simulink model "ieee80211n"  (Simulink 6.0)
settings: Solver=VariableStepDiscrete  StartTime=0.0  StopTime=inf  RelTol=1e-3
PreLoadFcn:
  | load IEEE80211n_init;
values from neighbouring files (symbols this model uses):
  params =     [IEEE80211n_init.mat]    (also in IEEE80211n_settings.m = p)
undefined symbols (not defined in the file or in its folder): magnitude
libraries: commblkintrlv2 x196, dspsigops x143, simulink x136, commdigbbndam2 x98, dspmtrx3 x96, dspsigattribs x69, dspstat3 x38, commutil2 x32, commsequence2 x26, commcnvcod2 x10, dspindex x9, dspmlti3 x8
(part 8 of 12)

== system ieee80211n/Demodbank/Demod_ss3/Demodulator 4 ==
  rxsig : Inport  Port=1  LatchInput=off
  mscale : Inport  Port=2  LatchInput=off
  Enable : EnablePort
  Bits Per Symbol : Constant  Value=ones(1, log2(modOrder))  VectorParams1D=off
  General Block Deinterleaver : commblkintrlv2/General Block Deinterleaver  elements=interleaverElements
  General Block Deinterleaver1 : S-Function  AncestorBlock=commblkintrlv2/General Block Deinterleaver  FunctionName=scominterl  Parameters=elements,method  mask(General Block Deinterleaver){elements=freqRotInterleaverElements}
      mask help: Reorder the elements of the input vector. y(elements) = u. The length of Elements must match the input signal width.
      mask init:
      | method = 2;
      | commblkinterl(elements);
      mask Help: helpview(commbhelp)
      mask Display: disp('Frequency\nRotation\nDeinterleaver')
  General Block Deinterleaver2 : commblkintrlv2/General Block Deinterleaver  elements=interleaverElements
  General Block Deinterleaver3 : S-Function  AncestorBlock=commblkintrlv2/General Block Deinterleaver  FunctionName=scominterl  Parameters=elements,method  mask(General Block Deinterleaver){elements=freqRotInterleaverElements}
      mask help: Reorder the elements of the input vector. y(elements) = u. The length of Elements must match the input signal width.
      mask init:
      | method = 2;
      | commblkinterl(elements);
      mask Help: helpview(commbhelp)
      mask Display: disp('Frequency\nRotation\nDeinterleaver')
  Matrix Deinterleaver : commblkintrlv2/Matrix Deinterleaver  Nrows=interleaverRows  Ncols=interleaverCols
  Matrix Deinterleaver1 : commblkintrlv2/Matrix Deinterleaver  Nrows=interleaverRows  Ncols=interleaverCols
  Matrix Multiply : Product  Multiplication=Matrix(*)
  Rectangular QAM Demodulator Baseband : commdigbbndam2/Rectangular QAM Demodulator Baseband  M=modOrder  OutType=Bit  Dec=Gray  PowType=Average Power  MinDist=2  AvgPow=1  PeakPow=1  Ph=0  numSamp=1
  Rectangular QAM Modulator Baseband1 : commdigbbndam2/Rectangular QAM Modulator Baseband  M=modOrder  InType=Bit  Enc=Gray  PowType=Average Power  MinDist=2  AvgPow=1  PeakPow=1  Ph=0  numSamp=1
  Reshape6 : simulink/Math Operations/Reshape  OutputDimensionality=Column vector  OutputDimensions=1600
  Sum : Sum  Inputs=|+-  SaturateOnIntegerOverflow=on
  Transpose : dspmtrx3/Transpose  Hermitian=off  overflowFlag=on
  Unipolar to Bipolar Converter2 : commutil2/Unipolar to Bipolar Converter  M=2  polarity=Negative
  rxdata : Outport  OutputWhenDisabled=reset  InitialOutput=0
  symerr : Outport  Port=2  OutputWhenDisabled=reset  InitialOutput=0
  mscale out : Outport  Port=3  OutputWhenDisabled=reset  InitialOutput=0
  wires:
  General Block Deinterleaver/1 -> Matrix Deinterleaver/1
  Matrix Deinterleaver/1 -> rxdata/1
  Sum/1 -> symerr/1
  Rectangular QAM Modulator Baseband1/1 -> Sum/1
  Unipolar to Bipolar Converter2/1 -> General Block Deinterleaver1/1
  rxsig/1 -> Sum/2, Rectangular QAM Demodulator Baseband/1
  Rectangular QAM Demodulator Baseband/1 -> Rectangular QAM Modulator Baseband1/1, Unipolar to Bipolar Converter2/1
  General Block Deinterleaver1/1 -> General Block Deinterleaver/1
  mscale/1 -> Matrix Multiply/1
  Matrix Multiply/1 -> Transpose/1
  Bits Per Symbol/1 -> Matrix Multiply/2
  Reshape6/1 -> General Block Deinterleaver3/1
  Transpose/1 -> Reshape6/1
  General Block Deinterleaver2/1 -> Matrix Deinterleaver1/1
  Matrix Deinterleaver1/1 -> mscale out/1
  General Block Deinterleaver3/1 -> General Block Deinterleaver2/1

== system ieee80211n/Demodbank/Demod_ss3/Demodulator 5 ==
  rxsig : Inport  Port=1  LatchInput=off
  mscale : Inport  Port=2  LatchInput=off
  Enable : EnablePort
  Bits Per Symbol : Constant  Value=ones(1, log2(modOrder))  VectorParams1D=off
  General Block Deinterleaver : commblkintrlv2/General Block Deinterleaver  elements=interleaverElements
  General Block Deinterleaver1 : S-Function  AncestorBlock=commblkintrlv2/General Block Deinterleaver  FunctionName=scominterl  Parameters=elements,method  mask(General Block Deinterleaver){elements=freqRotInterleaverElements}
      mask help: Reorder the elements of the input vector. y(elements) = u. The length of Elements must match the input signal width.
      mask init:
      | method = 2;
      | commblkinterl(elements);
      mask Help: helpview(commbhelp)
      mask Display: disp('Frequency\nRotation\nDeinterleaver')
  General Block Deinterleaver2 : commblkintrlv2/General Block Deinterleaver  elements=interleaverElements
  General Block Deinterleaver3 : S-Function  AncestorBlock=commblkintrlv2/General Block Deinterleaver  FunctionName=scominterl  Parameters=elements,method  mask(General Block Deinterleaver){elements=freqRotInterleaverElements}
      mask help: Reorder the elements of the input vector. y(elements) = u. The length of Elements must match the input signal width.
      mask init:
      | method = 2;
      | commblkinterl(elements);
      mask Help: helpview(commbhelp)
      mask Display: disp('Frequency\nRotation\nDeinterleaver')
  Matrix Deinterleaver : commblkintrlv2/Matrix Deinterleaver  Nrows=interleaverRows  Ncols=interleaverCols
  Matrix Deinterleaver1 : commblkintrlv2/Matrix Deinterleaver  Nrows=interleaverRows  Ncols=interleaverCols
  Matrix Multiply : Product  Multiplication=Matrix(*)
  Rectangular QAM Demodulator Baseband : commdigbbndam2/Rectangular QAM Demodulator Baseband  M=modOrder  OutType=Bit  Dec=Gray  PowType=Average Power  MinDist=2  AvgPow=1  PeakPow=1  Ph=0  numSamp=1
  Rectangular QAM Modulator Baseband1 : commdigbbndam2/Rectangular QAM Modulator Baseband  M=modOrder  InType=Bit  Enc=Gray  PowType=Average Power  MinDist=2  AvgPow=1  PeakPow=1  Ph=0  numSamp=1
  Reshape6 : simulink/Math Operations/Reshape  OutputDimensionality=Column vector  OutputDimensions=1600
  Sum : Sum  Inputs=|+-  SaturateOnIntegerOverflow=on
  Transpose : dspmtrx3/Transpose  Hermitian=off  overflowFlag=on
  Unipolar to Bipolar Converter2 : commutil2/Unipolar to Bipolar Converter  M=2  polarity=Negative
  rxdata : Outport  OutputWhenDisabled=reset  InitialOutput=0
  symerr : Outport  Port=2  OutputWhenDisabled=reset  InitialOutput=0
  mscale out : Outport  Port=3  OutputWhenDisabled=reset  InitialOutput=0
  wires:
  General Block Deinterleaver/1 -> Matrix Deinterleaver/1
  Matrix Deinterleaver/1 -> rxdata/1
  Sum/1 -> symerr/1
  Rectangular QAM Modulator Baseband1/1 -> Sum/1
  Unipolar to Bipolar Converter2/1 -> General Block Deinterleaver1/1
  rxsig/1 -> Sum/2, Rectangular QAM Demodulator Baseband/1
  Rectangular QAM Demodulator Baseband/1 -> Rectangular QAM Modulator Baseband1/1, Unipolar to Bipolar Converter2/1
  General Block Deinterleaver1/1 -> General Block Deinterleaver/1
  mscale/1 -> Matrix Multiply/1
  Matrix Multiply/1 -> Transpose/1
  Bits Per Symbol/1 -> Matrix Multiply/2
  Reshape6/1 -> General Block Deinterleaver3/1
  Transpose/1 -> Reshape6/1
  General Block Deinterleaver2/1 -> Matrix Deinterleaver1/1
  Matrix Deinterleaver1/1 -> mscale out/1
  General Block Deinterleaver3/1 -> General Block Deinterleaver2/1

== system ieee80211n/Demodbank/Demod_ss3/Demodulator 6 ==
  rxsig : Inport  Port=1  LatchInput=off
  mscale : Inport  Port=2  LatchInput=off
  Enable : EnablePort
  Bits Per Symbol : Constant  Value=ones(1, log2(modOrder))  VectorParams1D=off
  General Block Deinterleaver : commblkintrlv2/General Block Deinterleaver  elements=interleaverElements
  General Block Deinterleaver1 : S-Function  AncestorBlock=commblkintrlv2/General Block Deinterleaver  FunctionName=scominterl  Parameters=elements,method  mask(General Block Deinterleaver){elements=freqRotInterleaverElements}
      mask help: Reorder the elements of the input vector. y(elements) = u. The length of Elements must match the input signal width.
      mask init:
      | method = 2;
      | commblkinterl(elements);
      mask Help: helpview(commbhelp)
      mask Display: disp('Frequency\nRotation\nDeinterleaver')
  General Block Deinterleaver2 : commblkintrlv2/General Block Deinterleaver  elements=interleaverElements
  General Block Deinterleaver3 : S-Function  AncestorBlock=commblkintrlv2/General Block Deinterleaver  FunctionName=scominterl  Parameters=elements,method  mask(General Block Deinterleaver){elements=freqRotInterleaverElements}
      mask help: Reorder the elements of the input vector. y(elements) = u. The length of Elements must match the input signal width.
      mask init:
      | method = 2;
      | commblkinterl(elements);
      mask Help: helpview(commbhelp)
      mask Display: disp('Frequency\nRotation\nDeinterleaver')
  Matrix Deinterleaver : commblkintrlv2/Matrix Deinterleaver  Nrows=interleaverRows  Ncols=interleaverCols
  Matrix Deinterleaver1 : commblkintrlv2/Matrix Deinterleaver  Nrows=interleaverRows  Ncols=interleaverCols
  Matrix Multiply : Product  Multiplication=Matrix(*)
  Rectangular QAM Demodulator Baseband : commdigbbndam2/Rectangular QAM Demodulator Baseband  M=modOrder  OutType=Bit  Dec=Gray  PowType=Average Power  MinDist=2  AvgPow=1  PeakPow=1  Ph=0  numSamp=1
  Rectangular QAM Modulator Baseband1 : commdigbbndam2/Rectangular QAM Modulator Baseband  M=modOrder  InType=Bit  Enc=Gray  PowType=Average Power  MinDist=2  AvgPow=1  PeakPow=1  Ph=0  numSamp=1
  Reshape6 : simulink/Math Operations/Reshape  OutputDimensionality=Column vector  OutputDimensions=1600
  Sum : Sum  Inputs=|+-  SaturateOnIntegerOverflow=on
  Transpose : dspmtrx3/Transpose  Hermitian=off  overflowFlag=on
  Unipolar to Bipolar Converter2 : commutil2/Unipolar to Bipolar Converter  M=2  polarity=Negative
  rxdata : Outport  OutputWhenDisabled=reset  InitialOutput=0
  symerr : Outport  Port=2  OutputWhenDisabled=reset  InitialOutput=0
  mscale out : Outport  Port=3  OutputWhenDisabled=reset  InitialOutput=0
  wires:
  General Block Deinterleaver/1 -> Matrix Deinterleaver/1
  Matrix Deinterleaver/1 -> rxdata/1
  Sum/1 -> symerr/1
  Rectangular QAM Modulator Baseband1/1 -> Sum/1
  Unipolar to Bipolar Converter2/1 -> General Block Deinterleaver1/1
  rxsig/1 -> Sum/2, Rectangular QAM Demodulator Baseband/1
  Rectangular QAM Demodulator Baseband/1 -> Rectangular QAM Modulator Baseband1/1, Unipolar to Bipolar Converter2/1
  General Block Deinterleaver1/1 -> General Block Deinterleaver/1
  mscale/1 -> Matrix Multiply/1
  Matrix Multiply/1 -> Transpose/1
  Bits Per Symbol/1 -> Matrix Multiply/2
  Reshape6/1 -> General Block Deinterleaver3/1
  Transpose/1 -> Reshape6/1
  General Block Deinterleaver2/1 -> Matrix Deinterleaver1/1
  Matrix Deinterleaver1/1 -> mscale out/1
  General Block Deinterleaver3/1 -> General Block Deinterleaver2/1

== system ieee80211n/Demodbank/Demod_ss3/Demodulator 7 ==
  rxsig : Inport  Port=1  LatchInput=off
  mscale : Inport  Port=2  LatchInput=off
  Enable : EnablePort
  Bits Per Symbol : Constant  Value=ones(1, log2(modOrder))  VectorParams1D=off
  General Block Deinterleaver : commblkintrlv2/General Block Deinterleaver  elements=interleaverElements
  General Block Deinterleaver1 : S-Function  AncestorBlock=commblkintrlv2/General Block Deinterleaver  FunctionName=scominterl  Parameters=elements,method  mask(General Block Deinterleaver){elements=freqRotInterleaverElements}
      mask help: Reorder the elements of the input vector. y(elements) = u. The length of Elements must match the input signal width.
      mask init:
      | method = 2;
      | commblkinterl(elements);
      mask Help: helpview(commbhelp)
      mask Display: disp('Frequency\nRotation\nDeinterleaver')
  General Block Deinterleaver2 : commblkintrlv2/General Block Deinterleaver  elements=interleaverElements
  General Block Deinterleaver3 : S-Function  AncestorBlock=commblkintrlv2/General Block Deinterleaver  FunctionName=scominterl  Parameters=elements,method  mask(General Block Deinterleaver){elements=freqRotInterleaverElements}
      mask help: Reorder the elements of the input vector. y(elements) = u. The length of Elements must match the input signal width.
      mask init:
      | method = 2;
      | commblkinterl(elements);
      mask Help: helpview(commbhelp)
      mask Display: disp('Frequency\nRotation\nDeinterleaver')
  Matrix Deinterleaver : commblkintrlv2/Matrix Deinterleaver  Nrows=interleaverRows  Ncols=interleaverCols
  Matrix Deinterleaver1 : commblkintrlv2/Matrix Deinterleaver  Nrows=interleaverRows  Ncols=interleaverCols
  Matrix Multiply : Product  Multiplication=Matrix(*)
  Rectangular QAM Demodulator Baseband : commdigbbndam2/Rectangular QAM Demodulator Baseband  M=modOrder  OutType=Bit  Dec=Gray  PowType=Average Power  MinDist=2  AvgPow=1  PeakPow=1  Ph=0  numSamp=1
  Rectangular QAM Modulator Baseband1 : commdigbbndam2/Rectangular QAM Modulator Baseband  M=modOrder  InType=Bit  Enc=Gray  PowType=Average Power  MinDist=2  AvgPow=1  PeakPow=1  Ph=0  numSamp=1
  Reshape6 : simulink/Math Operations/Reshape  OutputDimensionality=Column vector  OutputDimensions=1600
  Sum : Sum  Inputs=|+-  SaturateOnIntegerOverflow=on
  Transpose : dspmtrx3/Transpose  Hermitian=off  overflowFlag=on
  Unipolar to Bipolar Converter2 : commutil2/Unipolar to Bipolar Converter  M=2  polarity=Negative
  rxdata : Outport  OutputWhenDisabled=reset  InitialOutput=0
  symerr : Outport  Port=2  OutputWhenDisabled=reset  InitialOutput=0
  mscale out : Outport  Port=3  OutputWhenDisabled=reset  InitialOutput=0
  wires:
  General Block Deinterleaver/1 -> Matrix Deinterleaver/1
  Matrix Deinterleaver/1 -> rxdata/1
  Sum/1 -> symerr/1
  Rectangular QAM Modulator Baseband1/1 -> Sum/1
  Unipolar to Bipolar Converter2/1 -> General Block Deinterleaver1/1
  rxsig/1 -> Sum/2, Rectangular QAM Demodulator Baseband/1
  Rectangular QAM Demodulator Baseband/1 -> Rectangular QAM Modulator Baseband1/1, Unipolar to Bipolar Converter2/1
  General Block Deinterleaver1/1 -> General Block Deinterleaver/1
  mscale/1 -> Matrix Multiply/1
  Matrix Multiply/1 -> Transpose/1
  Bits Per Symbol/1 -> Matrix Multiply/2
  Reshape6/1 -> General Block Deinterleaver3/1
  Transpose/1 -> Reshape6/1
  General Block Deinterleaver2/1 -> Matrix Deinterleaver1/1
  Matrix Deinterleaver1/1 -> mscale out/1
  General Block Deinterleaver3/1 -> General Block Deinterleaver2/1

== system ieee80211n/Demodbank/Demod_ss3/Demodulator 8 ==
  rxsig : Inport  Port=1  LatchInput=off
  mscale : Inport  Port=2  LatchInput=off
  Enable : EnablePort
  Bits Per Symbol : Constant  Value=ones(1, log2(modOrder))  VectorParams1D=off
  General Block Deinterleaver : commblkintrlv2/General Block Deinterleaver  elements=interleaverElements
  General Block Deinterleaver1 : S-Function  AncestorBlock=commblkintrlv2/General Block Deinterleaver  FunctionName=scominterl  Parameters=elements,method  mask(General Block Deinterleaver){elements=freqRotInterleaverElements}
      mask help: Reorder the elements of the input vector. y(elements) = u. The length of Elements must match the input signal width.
      mask init:
      | method = 2;
      | commblkinterl(elements);
      mask Help: helpview(commbhelp)
      mask Display: disp('Frequency\nRotation\nDeinterleaver')
  General Block Deinterleaver2 : commblkintrlv2/General Block Deinterleaver  elements=interleaverElements
  General Block Deinterleaver3 : S-Function  AncestorBlock=commblkintrlv2/General Block Deinterleaver  FunctionName=scominterl  Parameters=elements,method  mask(General Block Deinterleaver){elements=freqRotInterleaverElements}
      mask help: Reorder the elements of the input vector. y(elements) = u. The length of Elements must match the input signal width.
      mask init:
      | method = 2;
      | commblkinterl(elements);
      mask Help: helpview(commbhelp)
      mask Display: disp('Frequency\nRotation\nDeinterleaver')
  Matrix Deinterleaver : commblkintrlv2/Matrix Deinterleaver  Nrows=interleaverRows  Ncols=interleaverCols
  Matrix Deinterleaver1 : commblkintrlv2/Matrix Deinterleaver  Nrows=interleaverRows  Ncols=interleaverCols
  Matrix Multiply : Product  Multiplication=Matrix(*)
  Rectangular QAM Demodulator Baseband : commdigbbndam2/Rectangular QAM Demodulator Baseband  M=modOrder  OutType=Bit  Dec=Gray  PowType=Average Power  MinDist=2  AvgPow=1  PeakPow=1  Ph=0  numSamp=1
  Rectangular QAM Modulator Baseband1 : commdigbbndam2/Rectangular QAM Modulator Baseband  M=modOrder  InType=Bit  Enc=Gray  PowType=Average Power  MinDist=2  AvgPow=1  PeakPow=1  Ph=0  numSamp=1
  Reshape6 : simulink/Math Operations/Reshape  OutputDimensionality=Column vector  OutputDimensions=1600
  Sum : Sum  Inputs=|+-  SaturateOnIntegerOverflow=on
  Transpose : dspmtrx3/Transpose  Hermitian=off  overflowFlag=on
  Unipolar to Bipolar Converter2 : commutil2/Unipolar to Bipolar Converter  M=2  polarity=Negative
  rxdata : Outport  OutputWhenDisabled=reset  InitialOutput=0
  symerr : Outport  Port=2  OutputWhenDisabled=reset  InitialOutput=0
  mscale out : Outport  Port=3  OutputWhenDisabled=reset  InitialOutput=0
  wires:
  General Block Deinterleaver/1 -> Matrix Deinterleaver/1
  Matrix Deinterleaver/1 -> rxdata/1
  Sum/1 -> symerr/1
  Rectangular QAM Modulator Baseband1/1 -> Sum/1
  Unipolar to Bipolar Converter2/1 -> General Block Deinterleaver1/1
  rxsig/1 -> Sum/2, Rectangular QAM Demodulator Baseband/1
  Rectangular QAM Demodulator Baseband/1 -> Rectangular QAM Modulator Baseband1/1, Unipolar to Bipolar Converter2/1
  General Block Deinterleaver1/1 -> General Block Deinterleaver/1
  mscale/1 -> Matrix Multiply/1
  Matrix Multiply/1 -> Transpose/1
  Bits Per Symbol/1 -> Matrix Multiply/2
  Reshape6/1 -> General Block Deinterleaver3/1
  Transpose/1 -> Reshape6/1
  General Block Deinterleaver2/1 -> Matrix Deinterleaver1/1
  Matrix Deinterleaver1/1 -> mscale out/1
  General Block Deinterleaver3/1 -> General Block Deinterleaver2/1

== system ieee80211n/Demodbank/Demod_ss4/Demodulator 1 ==
  rxsig : Inport  Port=1  LatchInput=off
  mscale : Inport  Port=2  LatchInput=off
  Enable : EnablePort
  Bits Per Symbol : Constant  Value=ones(1, log2(modOrder))  VectorParams1D=off
  General Block Deinterleaver : commblkintrlv2/General Block Deinterleaver  elements=interleaverElements
  General Block Deinterleaver1 : S-Function  AncestorBlock=commblkintrlv2/General Block Deinterleaver  FunctionName=scominterl  Parameters=elements,method  mask(General Block Deinterleaver){elements=freqRotInterleaverElements}
      mask help: Reorder the elements of the input vector. y(elements) = u. The length of Elements must match the input signal width.
      mask init:
      | method = 2;
      | commblkinterl(elements);
      mask Help: helpview(commbhelp)
      mask Display: disp('Frequency\nRotation\nDeinterleaver')
  General Block Deinterleaver2 : commblkintrlv2/General Block Deinterleaver  elements=interleaverElements
  General Block Deinterleaver3 : S-Function  AncestorBlock=commblkintrlv2/General Block Deinterleaver  FunctionName=scominterl  Parameters=elements,method  mask(General Block Deinterleaver){elements=freqRotInterleaverElements}
      mask help: Reorder the elements of the input vector. y(elements) = u. The length of Elements must match the input signal width.
      mask init:
      | method = 2;
      | commblkinterl(elements);
      mask Help: helpview(commbhelp)
      mask Display: disp('Frequency\nRotation\nDeinterleaver')
  Matrix Deinterleaver : commblkintrlv2/Matrix Deinterleaver  Nrows=interleaverRows  Ncols=interleaverCols
  Matrix Deinterleaver1 : commblkintrlv2/Matrix Deinterleaver  Nrows=interleaverRows  Ncols=interleaverCols
  Matrix Multiply : Product  Multiplication=Matrix(*)
  Rectangular QAM Demodulator Baseband : commdigbbndam2/Rectangular QAM Demodulator Baseband  M=modOrder  OutType=Bit  Dec=Gray  PowType=Average Power  MinDist=2  AvgPow=1  PeakPow=1  Ph=0  numSamp=1
  Rectangular QAM Modulator Baseband1 : commdigbbndam2/Rectangular QAM Modulator Baseband  M=modOrder  InType=Bit  Enc=Gray  PowType=Average Power  MinDist=2  AvgPow=1  PeakPow=1  Ph=0  numSamp=1
  Reshape6 : simulink/Math Operations/Reshape  OutputDimensionality=Column vector  OutputDimensions=1600
  Sum : Sum  Inputs=|+-  SaturateOnIntegerOverflow=on
  Transpose : dspmtrx3/Transpose  Hermitian=off  overflowFlag=on
  Unipolar to Bipolar Converter2 : commutil2/Unipolar to Bipolar Converter  M=2  polarity=Negative
  rxdata : Outport  OutputWhenDisabled=reset  InitialOutput=0
  symerr : Outport  Port=2  OutputWhenDisabled=reset  InitialOutput=0
  mscale out : Outport  Port=3  OutputWhenDisabled=reset  InitialOutput=0
  wires:
  General Block Deinterleaver/1 -> Matrix Deinterleaver/1
  Matrix Deinterleaver/1 -> rxdata/1
  Sum/1 -> symerr/1
  Rectangular QAM Modulator Baseband1/1 -> Sum/1
  Unipolar to Bipolar Converter2/1 -> General Block Deinterleaver1/1
  rxsig/1 -> Sum/2, Rectangular QAM Demodulator Baseband/1
  Rectangular QAM Demodulator Baseband/1 -> Rectangular QAM Modulator Baseband1/1, Unipolar to Bipolar Converter2/1
  General Block Deinterleaver1/1 -> General Block Deinterleaver/1
  mscale/1 -> Matrix Multiply/1
  Matrix Multiply/1 -> Transpose/1
  Bits Per Symbol/1 -> Matrix Multiply/2
  Reshape6/1 -> General Block Deinterleaver3/1
  Transpose/1 -> Reshape6/1
  General Block Deinterleaver2/1 -> Matrix Deinterleaver1/1
  Matrix Deinterleaver1/1 -> mscale out/1
  General Block Deinterleaver3/1 -> General Block Deinterleaver2/1

== system ieee80211n/Demodbank/Demod_ss4/Demodulator 2 ==
  rxsig : Inport  Port=1  LatchInput=off
  mscale : Inport  Port=2  LatchInput=off
  Enable : EnablePort
  Bits Per Symbol : Constant  Value=ones(1, log2(modOrder))  VectorParams1D=off
  General Block Deinterleaver : commblkintrlv2/General Block Deinterleaver  elements=interleaverElements
  General Block Deinterleaver1 : S-Function  AncestorBlock=commblkintrlv2/General Block Deinterleaver  FunctionName=scominterl  Parameters=elements,method  mask(General Block Deinterleaver){elements=freqRotInterleaverElements}
      mask help: Reorder the elements of the input vector. y(elements) = u. The length of Elements must match the input signal width.
      mask init:
      | method = 2;
      | commblkinterl(elements);
      mask Help: helpview(commbhelp)
      mask Display: disp('Frequency\nRotation\nDeinterleaver')
  General Block Deinterleaver2 : commblkintrlv2/General Block Deinterleaver  elements=interleaverElements
  General Block Deinterleaver3 : S-Function  AncestorBlock=commblkintrlv2/General Block Deinterleaver  FunctionName=scominterl  Parameters=elements,method  mask(General Block Deinterleaver){elements=freqRotInterleaverElements}
      mask help: Reorder the elements of the input vector. y(elements) = u. The length of Elements must match the input signal width.
      mask init:
      | method = 2;
      | commblkinterl(elements);
      mask Help: helpview(commbhelp)
      mask Display: disp('Frequency\nRotation\nDeinterleaver')
  Matrix Deinterleaver : commblkintrlv2/Matrix Deinterleaver  Nrows=interleaverRows  Ncols=interleaverCols
  Matrix Deinterleaver1 : commblkintrlv2/Matrix Deinterleaver  Nrows=interleaverRows  Ncols=interleaverCols
  Matrix Multiply : Product  Multiplication=Matrix(*)
  Rectangular QAM Demodulator Baseband : commdigbbndam2/Rectangular QAM Demodulator Baseband  M=modOrder  OutType=Bit  Dec=Gray  PowType=Average Power  MinDist=2  AvgPow=1  PeakPow=1  Ph=0  numSamp=1
  Rectangular QAM Modulator Baseband1 : commdigbbndam2/Rectangular QAM Modulator Baseband  M=modOrder  InType=Bit  Enc=Gray  PowType=Average Power  MinDist=2  AvgPow=1  PeakPow=1  Ph=0  numSamp=1
  Reshape6 : simulink/Math Operations/Reshape  OutputDimensionality=Column vector  OutputDimensions=1600
  Sum : Sum  Inputs=|+-  SaturateOnIntegerOverflow=on
  Transpose : dspmtrx3/Transpose  Hermitian=off  overflowFlag=on
  Unipolar to Bipolar Converter2 : commutil2/Unipolar to Bipolar Converter  M=2  polarity=Negative
  rxdata : Outport  OutputWhenDisabled=reset  InitialOutput=0
  symerr : Outport  Port=2  OutputWhenDisabled=reset  InitialOutput=0
  mscale out : Outport  Port=3  OutputWhenDisabled=reset  InitialOutput=0
  wires:
  General Block Deinterleaver/1 -> Matrix Deinterleaver/1
  Matrix Deinterleaver/1 -> rxdata/1
  Sum/1 -> symerr/1
  Rectangular QAM Modulator Baseband1/1 -> Sum/1
  Unipolar to Bipolar Converter2/1 -> General Block Deinterleaver1/1
  rxsig/1 -> Sum/2, Rectangular QAM Demodulator Baseband/1
  Rectangular QAM Demodulator Baseband/1 -> Rectangular QAM Modulator Baseband1/1, Unipolar to Bipolar Converter2/1
  General Block Deinterleaver1/1 -> General Block Deinterleaver/1
  mscale/1 -> Matrix Multiply/1
  Matrix Multiply/1 -> Transpose/1
  Bits Per Symbol/1 -> Matrix Multiply/2
  Reshape6/1 -> General Block Deinterleaver3/1
  Transpose/1 -> Reshape6/1
  General Block Deinterleaver2/1 -> Matrix Deinterleaver1/1
  Matrix Deinterleaver1/1 -> mscale out/1
  General Block Deinterleaver3/1 -> General Block Deinterleaver2/1

== system ieee80211n/Demodbank/Demod_ss4/Demodulator 3 ==
  rxsig : Inport  Port=1  LatchInput=off
  mscale : Inport  Port=2  LatchInput=off
  Enable : EnablePort
  Bits Per Symbol : Constant  Value=ones(1, log2(modOrder))  VectorParams1D=off
  General Block Deinterleaver : commblkintrlv2/General Block Deinterleaver  elements=interleaverElements
  General Block Deinterleaver1 : S-Function  AncestorBlock=commblkintrlv2/General Block Deinterleaver  FunctionName=scominterl  Parameters=elements,method  mask(General Block Deinterleaver){elements=freqRotInterleaverElements}
      mask help: Reorder the elements of the input vector. y(elements) = u. The length of Elements must match the input signal width.
      mask init:
      | method = 2;
      | commblkinterl(elements);
      mask Help: helpview(commbhelp)
      mask Display: disp('Frequency\nRotation\nDeinterleaver')
  General Block Deinterleaver2 : commblkintrlv2/General Block Deinterleaver  elements=interleaverElements
  General Block Deinterleaver3 : S-Function  AncestorBlock=commblkintrlv2/General Block Deinterleaver  FunctionName=scominterl  Parameters=elements,method  mask(General Block Deinterleaver){elements=freqRotInterleaverElements}
      mask help: Reorder the elements of the input vector. y(elements) = u. The length of Elements must match the input signal width.
      mask init:
      | method = 2;
      | commblkinterl(elements);
      mask Help: helpview(commbhelp)
      mask Display: disp('Frequency\nRotation\nDeinterleaver')
  Matrix Deinterleaver : commblkintrlv2/Matrix Deinterleaver  Nrows=interleaverRows  Ncols=interleaverCols
  Matrix Deinterleaver1 : commblkintrlv2/Matrix Deinterleaver  Nrows=interleaverRows  Ncols=interleaverCols
  Matrix Multiply : Product  Multiplication=Matrix(*)
  Rectangular QAM Demodulator Baseband : commdigbbndam2/Rectangular QAM Demodulator Baseband  M=modOrder  OutType=Bit  Dec=Gray  PowType=Average Power  MinDist=2  AvgPow=1  PeakPow=1  Ph=0  numSamp=1
  Rectangular QAM Modulator Baseband1 : commdigbbndam2/Rectangular QAM Modulator Baseband  M=modOrder  InType=Bit  Enc=Gray  PowType=Average Power  MinDist=2  AvgPow=1  PeakPow=1  Ph=0  numSamp=1
  Reshape6 : simulink/Math Operations/Reshape  OutputDimensionality=Column vector  OutputDimensions=1600
  Sum : Sum  Inputs=|+-  SaturateOnIntegerOverflow=on
  Transpose : dspmtrx3/Transpose  Hermitian=off  overflowFlag=on
  Unipolar to Bipolar Converter2 : commutil2/Unipolar to Bipolar Converter  M=2  polarity=Negative
  rxdata : Outport  OutputWhenDisabled=reset  InitialOutput=0
  symerr : Outport  Port=2  OutputWhenDisabled=reset  InitialOutput=0
  mscale out : Outport  Port=3  OutputWhenDisabled=reset  InitialOutput=0
  wires:
  General Block Deinterleaver/1 -> Matrix Deinterleaver/1
  Matrix Deinterleaver/1 -> rxdata/1
  Sum/1 -> symerr/1
  Rectangular QAM Modulator Baseband1/1 -> Sum/1
  Unipolar to Bipolar Converter2/1 -> General Block Deinterleaver1/1
  rxsig/1 -> Sum/2, Rectangular QAM Demodulator Baseband/1
  Rectangular QAM Demodulator Baseband/1 -> Rectangular QAM Modulator Baseband1/1, Unipolar to Bipolar Converter2/1
  General Block Deinterleaver1/1 -> General Block Deinterleaver/1
  mscale/1 -> Matrix Multiply/1
  Matrix Multiply/1 -> Transpose/1
  Bits Per Symbol/1 -> Matrix Multiply/2
  Reshape6/1 -> General Block Deinterleaver3/1
  Transpose/1 -> Reshape6/1
  General Block Deinterleaver2/1 -> Matrix Deinterleaver1/1
  Matrix Deinterleaver1/1 -> mscale out/1
  General Block Deinterleaver3/1 -> General Block Deinterleaver2/1

== system ieee80211n/Demodbank/Demod_ss4/Demodulator 4 ==
  rxsig : Inport  Port=1  LatchInput=off
  mscale : Inport  Port=2  LatchInput=off
  Enable : EnablePort
  Bits Per Symbol : Constant  Value=ones(1, log2(modOrder))  VectorParams1D=off
  General Block Deinterleaver : commblkintrlv2/General Block Deinterleaver  elements=interleaverElements
  General Block Deinterleaver1 : S-Function  AncestorBlock=commblkintrlv2/General Block Deinterleaver  FunctionName=scominterl  Parameters=elements,method  mask(General Block Deinterleaver){elements=freqRotInterleaverElements}
      mask help: Reorder the elements of the input vector. y(elements) = u. The length of Elements must match the input signal width.
      mask init:
      | method = 2;
      | commblkinterl(elements);
      mask Help: helpview(commbhelp)
      mask Display: disp('Frequency\nRotation\nDeinterleaver')
  General Block Deinterleaver2 : commblkintrlv2/General Block Deinterleaver  elements=interleaverElements
  General Block Deinterleaver3 : S-Function  AncestorBlock=commblkintrlv2/General Block Deinterleaver  FunctionName=scominterl  Parameters=elements,method  mask(General Block Deinterleaver){elements=freqRotInterleaverElements}
      mask help: Reorder the elements of the input vector. y(elements) = u. The length of Elements must match the input signal width.
      mask init:
      | method = 2;
      | commblkinterl(elements);
      mask Help: helpview(commbhelp)
      mask Display: disp('Frequency\nRotation\nDeinterleaver')
  Matrix Deinterleaver : commblkintrlv2/Matrix Deinterleaver  Nrows=interleaverRows  Ncols=interleaverCols
  Matrix Deinterleaver1 : commblkintrlv2/Matrix Deinterleaver  Nrows=interleaverRows  Ncols=interleaverCols
  Matrix Multiply : Product  Multiplication=Matrix(*)
  Rectangular QAM Demodulator Baseband : commdigbbndam2/Rectangular QAM Demodulator Baseband  M=modOrder  OutType=Bit  Dec=Gray  PowType=Average Power  MinDist=2  AvgPow=1  PeakPow=1  Ph=0  numSamp=1
  Rectangular QAM Modulator Baseband1 : commdigbbndam2/Rectangular QAM Modulator Baseband  M=modOrder  InType=Bit  Enc=Gray  PowType=Average Power  MinDist=2  AvgPow=1  PeakPow=1  Ph=0  numSamp=1
  Reshape6 : simulink/Math Operations/Reshape  OutputDimensionality=Column vector  OutputDimensions=1600
  Sum : Sum  Inputs=|+-  SaturateOnIntegerOverflow=on
  Transpose : dspmtrx3/Transpose  Hermitian=off  overflowFlag=on
  Unipolar to Bipolar Converter2 : commutil2/Unipolar to Bipolar Converter  M=2  polarity=Negative
  rxdata : Outport  OutputWhenDisabled=reset  InitialOutput=0
  symerr : Outport  Port=2  OutputWhenDisabled=reset  InitialOutput=0
  mscale out : Outport  Port=3  OutputWhenDisabled=reset  InitialOutput=0
  wires:
  General Block Deinterleaver/1 -> Matrix Deinterleaver/1
  Matrix Deinterleaver/1 -> rxdata/1
  Sum/1 -> symerr/1
  Rectangular QAM Modulator Baseband1/1 -> Sum/1
  Unipolar to Bipolar Converter2/1 -> General Block Deinterleaver1/1
  rxsig/1 -> Sum/2, Rectangular QAM Demodulator Baseband/1
  Rectangular QAM Demodulator Baseband/1 -> Rectangular QAM Modulator Baseband1/1, Unipolar to Bipolar Converter2/1
  General Block Deinterleaver1/1 -> General Block Deinterleaver/1
  mscale/1 -> Matrix Multiply/1
  Matrix Multiply/1 -> Transpose/1
  Bits Per Symbol/1 -> Matrix Multiply/2
  Reshape6/1 -> General Block Deinterleaver3/1
  Transpose/1 -> Reshape6/1
  General Block Deinterleaver2/1 -> Matrix Deinterleaver1/1
  Matrix Deinterleaver1/1 -> mscale out/1
  General Block Deinterleaver3/1 -> General Block Deinterleaver2/1

== system ieee80211n/Demodbank/Demod_ss4/Demodulator 5 ==
  rxsig : Inport  Port=1  LatchInput=off
  mscale : Inport  Port=2  LatchInput=off
  Enable : EnablePort
  Bits Per Symbol : Constant  Value=ones(1, log2(modOrder))  VectorParams1D=off
  General Block Deinterleaver : commblkintrlv2/General Block Deinterleaver  elements=interleaverElements
  General Block Deinterleaver1 : S-Function  AncestorBlock=commblkintrlv2/General Block Deinterleaver  FunctionName=scominterl  Parameters=elements,method  mask(General Block Deinterleaver){elements=freqRotInterleaverElements}
      mask help: Reorder the elements of the input vector. y(elements) = u. The length of Elements must match the input signal width.
      mask init:
      | method = 2;
      | commblkinterl(elements);
      mask Help: helpview(commbhelp)
      mask Display: disp('Frequency\nRotation\nDeinterleaver')
  General Block Deinterleaver2 : commblkintrlv2/General Block Deinterleaver  elements=interleaverElements
  General Block Deinterleaver3 : S-Function  AncestorBlock=commblkintrlv2/General Block Deinterleaver  FunctionName=scominterl  Parameters=elements,method  mask(General Block Deinterleaver){elements=freqRotInterleaverElements}
      mask help: Reorder the elements of the input vector. y(elements) = u. The length of Elements must match the input signal width.
      mask init:
      | method = 2;
      | commblkinterl(elements);
      mask Help: helpview(commbhelp)
      mask Display: disp('Frequency\nRotation\nDeinterleaver')
  Matrix Deinterleaver : commblkintrlv2/Matrix Deinterleaver  Nrows=interleaverRows  Ncols=interleaverCols
  Matrix Deinterleaver1 : commblkintrlv2/Matrix Deinterleaver  Nrows=interleaverRows  Ncols=interleaverCols
  Matrix Multiply : Product  Multiplication=Matrix(*)
  Rectangular QAM Demodulator Baseband : commdigbbndam2/Rectangular QAM Demodulator Baseband  M=modOrder  OutType=Bit  Dec=Gray  PowType=Average Power  MinDist=2  AvgPow=1  PeakPow=1  Ph=0  numSamp=1
  Rectangular QAM Modulator Baseband1 : commdigbbndam2/Rectangular QAM Modulator Baseband  M=modOrder  InType=Bit  Enc=Gray  PowType=Average Power  MinDist=2  AvgPow=1  PeakPow=1  Ph=0  numSamp=1
  Reshape6 : simulink/Math Operations/Reshape  OutputDimensionality=Column vector  OutputDimensions=1600
  Sum : Sum  Inputs=|+-  SaturateOnIntegerOverflow=on
  Transpose : dspmtrx3/Transpose  Hermitian=off  overflowFlag=on
  Unipolar to Bipolar Converter2 : commutil2/Unipolar to Bipolar Converter  M=2  polarity=Negative
  rxdata : Outport  OutputWhenDisabled=reset  InitialOutput=0
  symerr : Outport  Port=2  OutputWhenDisabled=reset  InitialOutput=0
  mscale out : Outport  Port=3  OutputWhenDisabled=reset  InitialOutput=0
  wires:
  General Block Deinterleaver/1 -> Matrix Deinterleaver/1
  Matrix Deinterleaver/1 -> rxdata/1
  Sum/1 -> symerr/1
  Rectangular QAM Modulator Baseband1/1 -> Sum/1
  Unipolar to Bipolar Converter2/1 -> General Block Deinterleaver1/1
  rxsig/1 -> Sum/2, Rectangular QAM Demodulator Baseband/1
  Rectangular QAM Demodulator Baseband/1 -> Rectangular QAM Modulator Baseband1/1, Unipolar to Bipolar Converter2/1
  General Block Deinterleaver1/1 -> General Block Deinterleaver/1
  mscale/1 -> Matrix Multiply/1
  Matrix Multiply/1 -> Transpose/1
  Bits Per Symbol/1 -> Matrix Multiply/2
  Reshape6/1 -> General Block Deinterleaver3/1
  Transpose/1 -> Reshape6/1
  General Block Deinterleaver2/1 -> Matrix Deinterleaver1/1
  Matrix Deinterleaver1/1 -> mscale out/1
  General Block Deinterleaver3/1 -> General Block Deinterleaver2/1

== system ieee80211n/Demodbank/Demod_ss4/Demodulator 6 ==
  rxsig : Inport  Port=1  LatchInput=off
  mscale : Inport  Port=2  LatchInput=off
  Enable : EnablePort
  Bits Per Symbol : Constant  Value=ones(1, log2(modOrder))  VectorParams1D=off
  General Block Deinterleaver : commblkintrlv2/General Block Deinterleaver  elements=interleaverElements
  General Block Deinterleaver1 : S-Function  AncestorBlock=commblkintrlv2/General Block Deinterleaver  FunctionName=scominterl  Parameters=elements,method  mask(General Block Deinterleaver){elements=freqRotInterleaverElements}
      mask help: Reorder the elements of the input vector. y(elements) = u. The length of Elements must match the input signal width.
      mask init:
      | method = 2;
      | commblkinterl(elements);
      mask Help: helpview(commbhelp)
      mask Display: disp('Frequency\nRotation\nDeinterleaver')
  General Block Deinterleaver2 : commblkintrlv2/General Block Deinterleaver  elements=interleaverElements
  General Block Deinterleaver3 : S-Function  AncestorBlock=commblkintrlv2/General Block Deinterleaver  FunctionName=scominterl  Parameters=elements,method  mask(General Block Deinterleaver){elements=freqRotInterleaverElements}
      mask help: Reorder the elements of the input vector. y(elements) = u. The length of Elements must match the input signal width.
      mask init:
      | method = 2;
      | commblkinterl(elements);
      mask Help: helpview(commbhelp)
      mask Display: disp('Frequency\nRotation\nDeinterleaver')
  Matrix Deinterleaver : commblkintrlv2/Matrix Deinterleaver  Nrows=interleaverRows  Ncols=interleaverCols
  Matrix Deinterleaver1 : commblkintrlv2/Matrix Deinterleaver  Nrows=interleaverRows  Ncols=interleaverCols
  Matrix Multiply : Product  Multiplication=Matrix(*)
  Rectangular QAM Demodulator Baseband : commdigbbndam2/Rectangular QAM Demodulator Baseband  M=modOrder  OutType=Bit  Dec=Gray  PowType=Average Power  MinDist=2  AvgPow=1  PeakPow=1  Ph=0  numSamp=1
  Rectangular QAM Modulator Baseband1 : commdigbbndam2/Rectangular QAM Modulator Baseband  M=modOrder  InType=Bit  Enc=Gray  PowType=Average Power  MinDist=2  AvgPow=1  PeakPow=1  Ph=0  numSamp=1
  Reshape6 : simulink/Math Operations/Reshape  OutputDimensionality=Column vector  OutputDimensions=1600
  Sum : Sum  Inputs=|+-  SaturateOnIntegerOverflow=on
  Transpose : dspmtrx3/Transpose  Hermitian=off  overflowFlag=on
  Unipolar to Bipolar Converter2 : commutil2/Unipolar to Bipolar Converter  M=2  polarity=Negative
  rxdata : Outport  OutputWhenDisabled=reset  InitialOutput=0
  symerr : Outport  Port=2  OutputWhenDisabled=reset  InitialOutput=0
  mscale out : Outport  Port=3  OutputWhenDisabled=reset  InitialOutput=0
  wires:
  General Block Deinterleaver/1 -> Matrix Deinterleaver/1
  Matrix Deinterleaver/1 -> rxdata/1
  Sum/1 -> symerr/1
  Rectangular QAM Modulator Baseband1/1 -> Sum/1
  Unipolar to Bipolar Converter2/1 -> General Block Deinterleaver1/1
  rxsig/1 -> Sum/2, Rectangular QAM Demodulator Baseband/1
  Rectangular QAM Demodulator Baseband/1 -> Rectangular QAM Modulator Baseband1/1, Unipolar to Bipolar Converter2/1
  General Block Deinterleaver1/1 -> General Block Deinterleaver/1
  mscale/1 -> Matrix Multiply/1
  Matrix Multiply/1 -> Transpose/1
  Bits Per Symbol/1 -> Matrix Multiply/2
  Reshape6/1 -> General Block Deinterleaver3/1
  Transpose/1 -> Reshape6/1
  General Block Deinterleaver2/1 -> Matrix Deinterleaver1/1
  Matrix Deinterleaver1/1 -> mscale out/1
  General Block Deinterleaver3/1 -> General Block Deinterleaver2/1

== system ieee80211n/Demodbank/Demod_ss4/Demodulator 7 ==
  rxsig : Inport  Port=1  LatchInput=off
  mscale : Inport  Port=2  LatchInput=off
  Enable : EnablePort
  Bits Per Symbol : Constant  Value=ones(1, log2(modOrder))  VectorParams1D=off
  General Block Deinterleaver : commblkintrlv2/General Block Deinterleaver  elements=interleaverElements
  General Block Deinterleaver1 : S-Function  AncestorBlock=commblkintrlv2/General Block Deinterleaver  FunctionName=scominterl  Parameters=elements,method  mask(General Block Deinterleaver){elements=freqRotInterleaverElements}
      mask help: Reorder the elements of the input vector. y(elements) = u. The length of Elements must match the input signal width.
      mask init:
      | method = 2;
      | commblkinterl(elements);
      mask Help: helpview(commbhelp)
      mask Display: disp('Frequency\nRotation\nDeinterleaver')
  General Block Deinterleaver2 : commblkintrlv2/General Block Deinterleaver  elements=interleaverElements
  General Block Deinterleaver3 : S-Function  AncestorBlock=commblkintrlv2/General Block Deinterleaver  FunctionName=scominterl  Parameters=elements,method  mask(General Block Deinterleaver){elements=freqRotInterleaverElements}
      mask help: Reorder the elements of the input vector. y(elements) = u. The length of Elements must match the input signal width.
      mask init:
      | method = 2;
      | commblkinterl(elements);
      mask Help: helpview(commbhelp)
      mask Display: disp('Frequency\nRotation\nDeinterleaver')
  Matrix Deinterleaver : commblkintrlv2/Matrix Deinterleaver  Nrows=interleaverRows  Ncols=interleaverCols
  Matrix Deinterleaver1 : commblkintrlv2/Matrix Deinterleaver  Nrows=interleaverRows  Ncols=interleaverCols
  Matrix Multiply : Product  Multiplication=Matrix(*)
  Rectangular QAM Demodulator Baseband : commdigbbndam2/Rectangular QAM Demodulator Baseband  M=modOrder  OutType=Bit  Dec=Gray  PowType=Average Power  MinDist=2  AvgPow=1  PeakPow=1  Ph=0  numSamp=1
  Rectangular QAM Modulator Baseband1 : commdigbbndam2/Rectangular QAM Modulator Baseband  M=modOrder  InType=Bit  Enc=Gray  PowType=Average Power  MinDist=2  AvgPow=1  PeakPow=1  Ph=0  numSamp=1
  Reshape6 : simulink/Math Operations/Reshape  OutputDimensionality=Column vector  OutputDimensions=1600
  Sum : Sum  Inputs=|+-  SaturateOnIntegerOverflow=on
  Transpose : dspmtrx3/Transpose  Hermitian=off  overflowFlag=on
  Unipolar to Bipolar Converter2 : commutil2/Unipolar to Bipolar Converter  M=2  polarity=Negative
  rxdata : Outport  OutputWhenDisabled=reset  InitialOutput=0
  symerr : Outport  Port=2  OutputWhenDisabled=reset  InitialOutput=0
  mscale out : Outport  Port=3  OutputWhenDisabled=reset  InitialOutput=0
  wires:
  General Block Deinterleaver/1 -> Matrix Deinterleaver/1
  Matrix Deinterleaver/1 -> rxdata/1
  Sum/1 -> symerr/1
  Rectangular QAM Modulator Baseband1/1 -> Sum/1
  Unipolar to Bipolar Converter2/1 -> General Block Deinterleaver1/1
  rxsig/1 -> Sum/2, Rectangular QAM Demodulator Baseband/1
  Rectangular QAM Demodulator Baseband/1 -> Rectangular QAM Modulator Baseband1/1, Unipolar to Bipolar Converter2/1
  General Block Deinterleaver1/1 -> General Block Deinterleaver/1
  mscale/1 -> Matrix Multiply/1
  Matrix Multiply/1 -> Transpose/1
  Bits Per Symbol/1 -> Matrix Multiply/2
  Reshape6/1 -> General Block Deinterleaver3/1
  Transpose/1 -> Reshape6/1
  General Block Deinterleaver2/1 -> Matrix Deinterleaver1/1
  Matrix Deinterleaver1/1 -> mscale out/1
  General Block Deinterleaver3/1 -> General Block Deinterleaver2/1

== system ieee80211n/Demodbank/Demod_ss4/Demodulator 8 ==
  rxsig : Inport  Port=1  LatchInput=off
  mscale : Inport  Port=2  LatchInput=off
  Enable : EnablePort
  Bits Per Symbol : Constant  Value=ones(1, log2(modOrder))  VectorParams1D=off
  General Block Deinterleaver : commblkintrlv2/General Block Deinterleaver  elements=interleaverElements
  General Block Deinterleaver1 : S-Function  AncestorBlock=commblkintrlv2/General Block Deinterleaver  FunctionName=scominterl  Parameters=elements,method  mask(General Block Deinterleaver){elements=freqRotInterleaverElements}
      mask help: Reorder the elements of the input vector. y(elements) = u. The length of Elements must match the input signal width.
      mask init:
      | method = 2;
      | commblkinterl(elements);
      mask Help: helpview(commbhelp)
      mask Display: disp('Frequency\nRotation\nDeinterleaver')
  General Block Deinterleaver2 : commblkintrlv2/General Block Deinterleaver  elements=interleaverElements
  General Block Deinterleaver3 : S-Function  AncestorBlock=commblkintrlv2/General Block Deinterleaver  FunctionName=scominterl  Parameters=elements,method  mask(General Block Deinterleaver){elements=freqRotInterleaverElements}
      mask help: Reorder the elements of the input vector. y(elements) = u. The length of Elements must match the input signal width.
      mask init:
      | method = 2;
      | commblkinterl(elements);
      mask Help: helpview(commbhelp)
      mask Display: disp('Frequency\nRotation\nDeinterleaver')
  Matrix Deinterleaver : commblkintrlv2/Matrix Deinterleaver  Nrows=interleaverRows  Ncols=interleaverCols
  Matrix Deinterleaver1 : commblkintrlv2/Matrix Deinterleaver  Nrows=interleaverRows  Ncols=interleaverCols
  Matrix Multiply : Product  Multiplication=Matrix(*)
  Rectangular QAM Demodulator Baseband : commdigbbndam2/Rectangular QAM Demodulator Baseband  M=modOrder  OutType=Bit  Dec=Gray  PowType=Average Power  MinDist=2  AvgPow=1  PeakPow=1  Ph=0  numSamp=1
  Rectangular QAM Modulator Baseband1 : commdigbbndam2/Rectangular QAM Modulator Baseband  M=modOrder  InType=Bit  Enc=Gray  PowType=Average Power  MinDist=2  AvgPow=1  PeakPow=1  Ph=0  numSamp=1
  Reshape6 : simulink/Math Operations/Reshape  OutputDimensionality=Column vector  OutputDimensions=1600
  Sum : Sum  Inputs=|+-  SaturateOnIntegerOverflow=on
  Transpose : dspmtrx3/Transpose  Hermitian=off  overflowFlag=on
  Unipolar to Bipolar Converter2 : commutil2/Unipolar to Bipolar Converter  M=2  polarity=Negative
  rxdata : Outport  OutputWhenDisabled=reset  InitialOutput=0
  symerr : Outport  Port=2  OutputWhenDisabled=reset  InitialOutput=0
  mscale out : Outport  Port=3  OutputWhenDisabled=reset  InitialOutput=0
  wires:
  General Block Deinterleaver/1 -> Matrix Deinterleaver/1
  Matrix Deinterleaver/1 -> rxdata/1
  Sum/1 -> symerr/1
  Rectangular QAM Modulator Baseband1/1 -> Sum/1
  Unipolar to Bipolar Converter2/1 -> General Block Deinterleaver1/1
  rxsig/1 -> Sum/2, Rectangular QAM Demodulator Baseband/1
  Rectangular QAM Demodulator Baseband/1 -> Rectangular QAM Modulator Baseband1/1, Unipolar to Bipolar Converter2/1
  General Block Deinterleaver1/1 -> General Block Deinterleaver/1
  mscale/1 -> Matrix Multiply/1
  Matrix Multiply/1 -> Transpose/1
  Bits Per Symbol/1 -> Matrix Multiply/2
  Reshape6/1 -> General Block Deinterleaver3/1
  Transpose/1 -> Reshape6/1
  General Block Deinterleaver2/1 -> Matrix Deinterleaver1/1
  Matrix Deinterleaver1/1 -> mscale out/1
  General Block Deinterleaver3/1 -> General Block Deinterleaver2/1

== system ieee80211n/MIMODetection/Channel Estimation/ChannelEst1 ==
  trainsig : Inport  Port=1  LatchInput=off
  rxsig : Inport  Port=2  LatchInput=off
  Channel estimates : Subsystem
  Product1 : Product  Inputs=**  SaturateOnIntegerOverflow=on
  Remove DC component : Selector  InputType=Matrix  Elements=[1:26 27:]  Rows=[1:28 30:57]  Columns=-1  InputPortWidth=53
  Remove training DC component : Selector  InputType=Matrix  Elements=[1:26 27:]  Rows=[1:28 30:57]  Columns=-1  InputPortWidth=53
  Select training/data : S-Function  AncestorBlock=dspindex/Multiport Selector  FunctionName=sdspmultiportsel  Parameters=rowsOrCols, numOutports, flatIdxVect, flatLenVect, idxErrMode  mask(Multiport Selector){rowsOrCols=Columns, idxCellArray={params.OFDM_TotPreamblePerFrame-params.OFDM_HTLTF_SymPerFrame+1:params.OFDM_TotPreamblePerFrame}, idxErrMode=Clip Index}
      mask prompts: rowsOrCols "Select:"; idxCellArray "Indices to output:"; idxErrMode "Invalid index:"
      mask help: Output specified rows or columns to one or more output ports. The number of output ports is determined by the number of index vectors, each specified as a separate vector entry in a cell array. Indices are 1-based and need not be unique.
      mask init:
      | [numOutports, flatLenVect, flatIdxVect] = dspblkmultiportsel(idxCellArray);
      mask Help: web(dspbhelp);
      mask StyleString: popup(Rows|Columns),edit,popup(Clip Index|Clip and Warn|Generate Error)
      mask Display: disp(['Select\n' &1]);
  out : Outport
  wires:
  rxsig/1 -> Remove DC component/1
  Channel estimates/1(ch est) -> out/1
  trainsig/1 -> Remove training DC component/1
  Product1/1 -> Channel estimates/2(in)
  Select training/data/1 -> Product1/2
  Remove DC component/1 -> Select training/data/1
  Remove training DC component/1 -> Product1/1, Channel estimates/1(trn)
